simulink model "SMA_mass"  (R2018a)
settings: Solver=ode15s  StartTime=0.0  StopTime=30  MaxStep=0.01  RelTol=1e-6  EnableMultiTasking=on
InitFcn:
  | Parameter;
undefined symbols (not defined in the file or in its folder): bias
settings Model: Creator=Johannes  LastModifiedBy=Matthias
settings DataIOCC: LimitDataPoints=on  SaveFormat=Array  SignalLoggingSaveFormat=ModelDataLogs
settings OptimizationCC: LifeSpan=inf
settings DebuggingCC: UnderspecifiedInitializationDetection=Classic  MergeDetectMultiDrivingBlocksExec=none  SolverPrmCheckMsg=warning  MultiTaskDSMMsg=warning  MultiTaskCondExecSysMsg=none  SFUnexpectedBacktrackingDiag=warning  SFNoUnconditionalDefaultTransitionDiag=warning  SFExecutionAtInitializationDiag=none
settings HardwareCC: ProdBitPerPointer=32  ProdBitPerSizeT=32  ProdBitPerPtrDiffT=32  ProdLargestAtomicFloat=None  ProdIntDivRoundTo=Undefined  ProdEndianess=Unspecified  ProdWordSize=32  ProdHWDeviceType=32-bit Generic
settings ModelReferenceCC: PropagateSignalLabelsOutOfModel=off
settings CodeAppCC: StateflowObjectComments=on
settings GRTTargetCC: TargetLangStandard=C89/C90 (ANSI)  GeneratePreprocessorConditionals=Disable all
settings ConfigComp: CovMetricSettings=dw  CovHtmlReporting=on  CovSaveCumulativeToWorkspaceVar=on  CovSaveSingleToWorkspaceVar=on  CovExternalEMLEnable=off

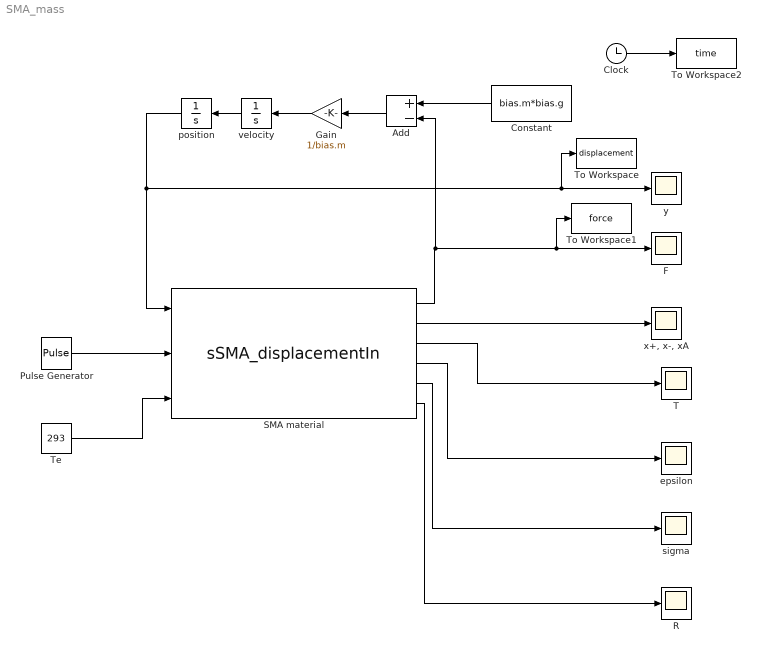
== system SMA_mass ==
  Add : Sum  Inputs=+-
  Clock : Clock
  Constant : Constant  Value=bias.m*bias.g
  F : Scope
  Gain : Gain  Gain=1/bias.m
  Pulse Generator : DiscretePulseGenerator  PulseType=Time based  Amplitude=0.4  Period=10  PulseWidth=5
  R : Scope
  SMA material : M-S-Function  FunctionName=sSMA_displacementIn  Parameters=params, initConds
      mask Display:
      | color('black');
      | patch(3*[-1 1 1 -1],1.1*[-1 -1 1 1],[1 1 1]);
      | patch([-1.6 -0.8],[-0.9 0.3],[0 0 0]);
      | patch([-0.8 1.2],[0.3 0.3],[0 0 0]);
      | patch([1.6 0.8],[0.9 -0.3],[0 0 0]);
      | patch([0.8 -1.2],[-0.3 -0.3],[0 0 0]);
      | disp('SMA');
      | 
      | color('blue');
      | port_label('input', 1, 'y [m]','texmode','on');
      | port_label('input', 2, 'J [W]','texmode','on');
      | port_label('input', 3, 'T_E [K]','texmode','on');
      | 
      | color('red');
      | port_label('output', 1, 'F [N]','texmode','on');
      | port_label('output', 2, 'x_+, x_-, x_A [-]','texmode','on');
      | port_label('output', 3, 'T [K]','texmode','on');
      | port_label('output', 4, '\epsilon [-]','texmode','on');
      | port_label('output', 5, '\sigma [Pa]','texmode','on');
      | port_label('output', 6, 'R [\Omega]','texmode','on');
  T : Scope
  Te : Constant  Value=293
  To Workspace : ToWorkspace  VariableName=displacement  SampleTime=-1
  To Workspace1 : ToWorkspace  VariableName=force  SampleTime=-1
  To Workspace2 : ToWorkspace  VariableName=time  SampleTime=-1
  epsilon : Scope
  position : Integrator  InitialCondition=bias.y0
  sigma : Scope
  velocity : Integrator  InitialCondition=bias.v0
  "x+, x-, xA" : Scope
  y : Scope
  wires:
  Pulse Generator/1 -> SMA material/2
  Te/1 -> SMA material/3
  SMA material/1 -> Add/2, To Workspace1/1, F/1
  SMA material/2 -> "x+, x-, xA"/1
  SMA material/3 -> T/1
  SMA material/4 -> epsilon/1
  SMA material/5 -> sigma/1
  SMA material/6 -> R/1
  Constant/1 -> Add/1
  Add/1 -> Gain/1
  velocity/1 -> position/1
  position/1 -> To Workspace/1, y/1, SMA material/1
  Gain/1 -> velocity/1
  Clock/1 -> To Workspace2/1
